simulink model "BD_PAR_AUTO_base_model"  (Simulink 10.3)
settings: Solver=ode1  StartTime=0.0  StopTime=max(cyc_mph(:,1))  FixedStep=1  MaxStep=1  RelTol=1e-3  AbsTol=1e-3
undefined symbols (not defined in the file): acc_dcdc_eff, acc_elec_eff, acc_elec_pwr, acc_mech_eff, acc_mech_pwr, acc_mech_trq, air_cp, amb_tmp, cs_charge_deplete_bool, cs_charge_trq, cs_electric_decel_spd, cs_electric_launch_spd_hi, cs_electric_launch_spd_lo, cs_hi_soc, cs_lo_soc, cs_min_trq_frac, cs_off_trq_frac, cyc_avg_time, cyc_cargo_mass, cyc_elevation_init, cyc_filter_bool, cyc_grade, cyc_mph, enable_sim_stop_distance, enable_sim_stop_max_spd, enable_sim_stop_speed, enable_sim_stop_time, enable_stop, enable_stop_fc, ess_cap_scale, ess_coulombic_eff, ess_init_soc, ess_max_ah_cap, ess_max_volts, ess_min_volts, ess_mod_airflow, ess_mod_cp, ess_mod_init_tmp, ess_module_mass, ess_module_num, ess_on, ess_r_chg, ess_r_dis, ess_res_scale_coef, ess_res_scale_fun, ess_set_tmp, ess_soc, ess_th_calc, ess_th_res_off, ess_th_res_on, ess_tmp, ess_voc, ex_calc, ex_cat_co_frac, ex_cat_ext_cp, ex_cat_ext_emisv, ex_cat_ext_init_tmp, ex_cat_ext_mass, ex_cat_ext_sarea, ex_cat_hc_frac ... (+168)
(part 12 of 15)

== system BD_PAR_AUTO_base_model/mechanical accessory loads <acc>/Mechanical Accessory Loads v2 <acc>/backward model/mechanical accessories (Nm)/Mechanical Accessories: Const Mech Var Elect/Elec Aux Loads 14V Pwr/FrontHVAC/Subsystem/Subsystem ==
  Constant1 : Constant  Value=0
  DurationOn1 : Subsystem  mask{ModelName=ModelName}
      mask prompts: ModelName "Auxiliary Load Model"
      mask init: same as BD_PAR_AUTO_base_model/electric acc loads <acc>/Electrical Accessory Loads v2 <acc>/backward model/electrical accessories (W)/Electrical Accessories: Time Variable/Elec Aux Loads 14V Pwr/ExternalLights/Subsystem/Subsystem/DurationOn1
  Hit  Crossing3 : HitCross  HitCrossingDirection=rising
  Hold Load On : RelationalOperator  Operator=<  RndMeth=Nearest  InputSameDT=on
  Hold Load On1 : RelationalOperator  RndMeth=Nearest  InputSameDT=on
  Load On : Logic  Operator=OR
  Memory5 : Memory  InitialCondition=eval('evalin(''base'',[''vinf.AuxLoads.'',ModelName,''.OnOffInfo.StartTime''])','0')
  Period1 : Subsystem  mask{ModelName=ModelName}
      mask prompts: ModelName "Auxiliary Load Model"
      mask init: same as BD_PAR_AUTO_base_model/electric acc loads <acc>/Electrical Accessory Loads v2 <acc>/backward model/electrical accessories (W)/Electrical Accessories: Time Variable/Elec Aux Loads 14V Pwr/ExternalLights/Subsystem/Subsystem/Period1
  Relational Operator1 : RelationalOperator  Operator=<=  RndMeth=Nearest  InputSameDT=on
  Relational Operator3 : RelationalOperator  Operator=>  RndMeth=Nearest  InputSameDT=on
  StartTime1 : Subsystem  mask{ModelName=ModelName}
      mask prompts: ModelName "Auxiliary Load Model"
      mask init: same as BD_PAR_AUTO_base_model/electric acc loads <acc>/Electrical Accessory Loads v2 <acc>/backward model/electrical accessories (W)/Electrical Accessories: Time Variable/Elec Aux Loads 14V Pwr/ExternalLights/Subsystem/Subsystem/StartTime1
  StartTime3 : Subsystem  mask{ModelName=ModelName}
      mask prompts: ModelName "Auxiliary Load Model"
      mask init: same as BD_PAR_AUTO_base_model/electric acc loads <acc>/Electrical Accessory Loads v2 <acc>/backward model/electrical accessories (W)/Electrical Accessories: Time Variable/Elec Aux Loads 14V Pwr/ExternalLights/Subsystem/Subsystem/StartTime1
  Sum1 : Sum  SaturateOnIntegerOverflow=on
  Sum3 : Sum  SaturateOnIntegerOverflow=on
  Switch1 : Switch  Threshold=.5
  Triggered Subsystem2 : Subsystem  TreatAsAtomicUnit=on  mask{ModelName=ModelName}
      mask prompts: ModelName "Load Name"
      mask init:
      | if (evalin('base',['isfield(vinf.AuxLoads.',ModelName,'.OnOffInfo,''StartTime'')'])); StartTime=evalin('base',['vinf.AuxLoads.',ModelName,'.OnOffInfo.StartTime']); else; StartTime=0;end
  Turn Load On : Logic  Operator=OR
  Reg Cycle On/Off : Outport
  wires:
  Memory5/1 -> Sum1/2, Sum3/2
  Sum3/1 -> Hold Load On1/2
  [time] -> Hold Load On1/1
  Turn Load On/1 -> Load On/1
  Hit  Crossing3/1 -> Turn Load On/1
  Hold Load On/1 -> Load On/2
  Hold Load On1/1 -> Turn Load On/2
  Load On/1 -> Switch1/3
  Sum1/1 -> Hold Load On/2
  [time] -> Hold Load On/1
  Relational Operator3/1 -> Hit  Crossing3/1
  [time] -> Relational Operator3/1
  StartTime1/1(Out1) -> Relational Operator3/2
  Triggered Subsystem2/1(last trig on time) -> Memory5/1
  [time] -> Triggered Subsystem2/1(time)
  Constant1/1 -> Switch1/1
  Relational Operator1/1 -> Switch1/2
  [time] -> Relational Operator1/1
  StartTime3/1(Out1) -> Relational Operator1/2
  Switch1/1 -> Reg Cycle On/Off/1, Triggered Subsystem2/Trigger
  Period1/1(Out1) -> Sum3/1
  DurationOn1/1(Out1) -> Sum1/1

== system BD_PAR_AUTO_base_model/mechanical accessory loads <acc>/Mechanical Accessory Loads v2 <acc>/backward model/mechanical accessories (Nm)/Mechanical Accessories: Const Mech Var Elect/Elec Aux Loads 14V Pwr/FrontHVAC/Subsystem/Subsystem1 ==
  Memory1 : Memory
  Memory3 : Memory
  Relational Operator1 : RelationalOperator  Operator=>  RndMeth=Nearest  InputSameDT=on
  Relational Operator2 : RelationalOperator  Operator=~=  RndMeth=Nearest  InputSameDT=on
  Sum : Sum  Inputs=+  SaturateOnIntegerOverflow=on
  ToggleTimes : Subsystem  mask{ModelName=ModelName}
      mask prompts: ModelName "Auxiliary Load Model"
      mask init: same as BD_PAR_AUTO_base_model/electric acc loads <acc>/Electrical Accessory Loads v2 <acc>/backward model/electrical accessories (W)/Electrical Accessories: Time Variable/Elec Aux Loads 14V Pwr/ExternalLights/Subsystem/Subsystem1/ToggleTimes
  Triggered Subsystem1 : Subsystem  TreatAsAtomicUnit=on  mask{ModelName=ModelName}
      mask prompts: ModelName "Load Name"
      mask init:
      | if (evalin('base',['isfield(vinf.AuxLoads.',ModelName,'.OnOffInfo,''InitialOn'')'])); InitialOn=evalin('base',['vinf.AuxLoads.',ModelName,'.OnOffInfo.InitialOn']);else;InitialOn=0;end
  Toggle On/Off : Outport
  wires:
  [time] -> Relational Operator1/1
  ToggleTimes/1(Out1) -> Relational Operator1/2
  Relational Operator1/1 -> Sum/1
  Sum/1 -> Memory1/1, Relational Operator2/1
  Relational Operator2/1 -> Triggered Subsystem1/Enable
  Triggered Subsystem1/1(Out1) -> Memory3/1, Toggle On/Off/1
  Memory3/1 -> Triggered Subsystem1/1(In1)
  Memory1/1 -> Relational Operator2/2

== system BD_PAR_AUTO_base_model/mechanical accessory loads <acc>/Mechanical Accessory Loads v2 <acc>/backward model/mechanical accessories (Nm)/Mechanical Accessories: Const Mech Var Elect/Elec Aux Loads 14V Pwr/FrontWipers/Subsystem/Subsystem ==
  Constant1 : Constant  Value=0
  DurationOn1 : Subsystem  mask{ModelName=ModelName}
      mask prompts: ModelName "Auxiliary Load Model"
      mask init: same as BD_PAR_AUTO_base_model/electric acc loads <acc>/Electrical Accessory Loads v2 <acc>/backward model/electrical accessories (W)/Electrical Accessories: Time Variable/Elec Aux Loads 14V Pwr/ExternalLights/Subsystem/Subsystem/DurationOn1
  Hit  Crossing3 : HitCross  HitCrossingDirection=rising
  Hold Load On : RelationalOperator  Operator=<  RndMeth=Nearest  InputSameDT=on
  Hold Load On1 : RelationalOperator  RndMeth=Nearest  InputSameDT=on
  Load On : Logic  Operator=OR
  Memory5 : Memory  InitialCondition=eval('evalin(''base'',[''vinf.AuxLoads.'',ModelName,''.OnOffInfo.StartTime''])','0')
  Period1 : Subsystem  mask{ModelName=ModelName}
      mask prompts: ModelName "Auxiliary Load Model"
      mask init: same as BD_PAR_AUTO_base_model/electric acc loads <acc>/Electrical Accessory Loads v2 <acc>/backward model/electrical accessories (W)/Electrical Accessories: Time Variable/Elec Aux Loads 14V Pwr/ExternalLights/Subsystem/Subsystem/Period1
  Relational Operator1 : RelationalOperator  Operator=<=  RndMeth=Nearest  InputSameDT=on
  Relational Operator3 : RelationalOperator  Operator=>  RndMeth=Nearest  InputSameDT=on
  StartTime1 : Subsystem  mask{ModelName=ModelName}
      mask prompts: ModelName "Auxiliary Load Model"
      mask init: same as BD_PAR_AUTO_base_model/electric acc loads <acc>/Electrical Accessory Loads v2 <acc>/backward model/electrical accessories (W)/Electrical Accessories: Time Variable/Elec Aux Loads 14V Pwr/ExternalLights/Subsystem/Subsystem/StartTime1
  StartTime3 : Subsystem  mask{ModelName=ModelName}
      mask prompts: ModelName "Auxiliary Load Model"
      mask init: same as BD_PAR_AUTO_base_model/electric acc loads <acc>/Electrical Accessory Loads v2 <acc>/backward model/electrical accessories (W)/Electrical Accessories: Time Variable/Elec Aux Loads 14V Pwr/ExternalLights/Subsystem/Subsystem/StartTime1
  Sum1 : Sum  SaturateOnIntegerOverflow=on
  Sum3 : Sum  SaturateOnIntegerOverflow=on
  Switch1 : Switch  Threshold=.5
  Triggered Subsystem2 : Subsystem  TreatAsAtomicUnit=on  mask{ModelName=ModelName}
      mask prompts: ModelName "Load Name"
      mask init:
      | if (evalin('base',['isfield(vinf.AuxLoads.',ModelName,'.OnOffInfo,''StartTime'')'])); StartTime=evalin('base',['vinf.AuxLoads.',ModelName,'.OnOffInfo.StartTime']); else; StartTime=0;end
  Turn Load On : Logic  Operator=OR
  Reg Cycle On/Off : Outport
  wires:
  Memory5/1 -> Sum1/2, Sum3/2
  Sum3/1 -> Hold Load On1/2
  [time] -> Hold Load On1/1
  Turn Load On/1 -> Load On/1
  Hit  Crossing3/1 -> Turn Load On/1
  Hold Load On/1 -> Load On/2
  Hold Load On1/1 -> Turn Load On/2
  Load On/1 -> Switch1/3
  Sum1/1 -> Hold Load On/2
  [time] -> Hold Load On/1
  Relational Operator3/1 -> Hit  Crossing3/1
  [time] -> Relational Operator3/1
  StartTime1/1(Out1) -> Relational Operator3/2
  Triggered Subsystem2/1(last trig on time) -> Memory5/1
  [time] -> Triggered Subsystem2/1(time)
  Constant1/1 -> Switch1/1
  Relational Operator1/1 -> Switch1/2
  [time] -> Relational Operator1/1
  StartTime3/1(Out1) -> Relational Operator1/2
  Switch1/1 -> Reg Cycle On/Off/1, Triggered Subsystem2/Trigger
  Period1/1(Out1) -> Sum3/1
  DurationOn1/1(Out1) -> Sum1/1

== system BD_PAR_AUTO_base_model/mechanical accessory loads <acc>/Mechanical Accessory Loads v2 <acc>/backward model/mechanical accessories (Nm)/Mechanical Accessories: Const Mech Var Elect/Elec Aux Loads 14V Pwr/FrontWipers/Subsystem/Subsystem1 ==
  Memory1 : Memory
  Memory3 : Memory
  Relational Operator1 : RelationalOperator  Operator=>  RndMeth=Nearest  InputSameDT=on
  Relational Operator2 : RelationalOperator  Operator=~=  RndMeth=Nearest  InputSameDT=on
  Sum : Sum  Inputs=+  SaturateOnIntegerOverflow=on
  ToggleTimes : Subsystem  mask{ModelName=ModelName}
      mask prompts: ModelName "Auxiliary Load Model"
      mask init: same as BD_PAR_AUTO_base_model/electric acc loads <acc>/Electrical Accessory Loads v2 <acc>/backward model/electrical accessories (W)/Electrical Accessories: Time Variable/Elec Aux Loads 14V Pwr/ExternalLights/Subsystem/Subsystem1/ToggleTimes
  Triggered Subsystem1 : Subsystem  TreatAsAtomicUnit=on  mask{ModelName=ModelName}
      mask prompts: ModelName "Load Name"
      mask init:
      | if (evalin('base',['isfield(vinf.AuxLoads.',ModelName,'.OnOffInfo,''InitialOn'')'])); InitialOn=evalin('base',['vinf.AuxLoads.',ModelName,'.OnOffInfo.InitialOn']);else;InitialOn=0;end
  Toggle On/Off : Outport
  wires:
  [time] -> Relational Operator1/1
  ToggleTimes/1(Out1) -> Relational Operator1/2
  Relational Operator1/1 -> Sum/1
  Sum/1 -> Memory1/1, Relational Operator2/1
  Relational Operator2/1 -> Triggered Subsystem1/Enable
  Triggered Subsystem1/1(Out1) -> Memory3/1, Toggle On/Off/1
  Memory3/1 -> Triggered Subsystem1/1(In1)
  Memory1/1 -> Relational Operator2/2

== system BD_PAR_AUTO_base_model/mechanical accessory loads <acc>/Mechanical Accessory Loads v2 <acc>/backward model/mechanical accessories (Nm)/Mechanical Accessories: Const Mech Var Elect/Elec Aux Loads 14V Pwr/HeatedSeats/Subsystem/Subsystem ==
  Constant1 : Constant  Value=0
  DurationOn1 : Subsystem  mask{ModelName=ModelName}
      mask prompts: ModelName "Auxiliary Load Model"
      mask init: same as BD_PAR_AUTO_base_model/electric acc loads <acc>/Electrical Accessory Loads v2 <acc>/backward model/electrical accessories (W)/Electrical Accessories: Time Variable/Elec Aux Loads 14V Pwr/ExternalLights/Subsystem/Subsystem/DurationOn1
  Hit  Crossing3 : HitCross  HitCrossingDirection=rising
  Hold Load On : RelationalOperator  Operator=<  RndMeth=Nearest  InputSameDT=on
  Hold Load On1 : RelationalOperator  RndMeth=Nearest  InputSameDT=on
  Load On : Logic  Operator=OR
  Memory5 : Memory  InitialCondition=eval('evalin(''base'',[''vinf.AuxLoads.'',ModelName,''.OnOffInfo.StartTime''])','0')
  Period1 : Subsystem  mask{ModelName=ModelName}
      mask prompts: ModelName "Auxiliary Load Model"
      mask init: same as BD_PAR_AUTO_base_model/electric acc loads <acc>/Electrical Accessory Loads v2 <acc>/backward model/electrical accessories (W)/Electrical Accessories: Time Variable/Elec Aux Loads 14V Pwr/ExternalLights/Subsystem/Subsystem/Period1
  Relational Operator1 : RelationalOperator  Operator=<=  RndMeth=Nearest  InputSameDT=on
  Relational Operator3 : RelationalOperator  Operator=>  RndMeth=Nearest  InputSameDT=on
  StartTime1 : Subsystem  mask{ModelName=ModelName}
      mask prompts: ModelName "Auxiliary Load Model"
      mask init: same as BD_PAR_AUTO_base_model/electric acc loads <acc>/Electrical Accessory Loads v2 <acc>/backward model/electrical accessories (W)/Electrical Accessories: Time Variable/Elec Aux Loads 14V Pwr/ExternalLights/Subsystem/Subsystem/StartTime1
  StartTime3 : Subsystem  mask{ModelName=ModelName}
      mask prompts: ModelName "Auxiliary Load Model"
      mask init: same as BD_PAR_AUTO_base_model/electric acc loads <acc>/Electrical Accessory Loads v2 <acc>/backward model/electrical accessories (W)/Electrical Accessories: Time Variable/Elec Aux Loads 14V Pwr/ExternalLights/Subsystem/Subsystem/StartTime1
  Sum1 : Sum  SaturateOnIntegerOverflow=on
  Sum3 : Sum  SaturateOnIntegerOverflow=on
  Switch1 : Switch  Threshold=.5
  Triggered Subsystem2 : Subsystem  TreatAsAtomicUnit=on  mask{ModelName=ModelName}
      mask prompts: ModelName "Load Name"
      mask init:
      | if (evalin('base',['isfield(vinf.AuxLoads.',ModelName,'.OnOffInfo,''StartTime'')'])); StartTime=evalin('base',['vinf.AuxLoads.',ModelName,'.OnOffInfo.StartTime']); else; StartTime=0;end
  Turn Load On : Logic  Operator=OR
  Reg Cycle On/Off : Outport
  wires:
  Memory5/1 -> Sum1/2, Sum3/2
  Sum3/1 -> Hold Load On1/2
  [time] -> Hold Load On1/1
  Turn Load On/1 -> Load On/1
  Hit  Crossing3/1 -> Turn Load On/1
  Hold Load On/1 -> Load On/2
  Hold Load On1/1 -> Turn Load On/2
  Load On/1 -> Switch1/3
  Sum1/1 -> Hold Load On/2
  [time] -> Hold Load On/1
  Relational Operator3/1 -> Hit  Crossing3/1
  [time] -> Relational Operator3/1
  StartTime1/1(Out1) -> Relational Operator3/2
  Triggered Subsystem2/1(last trig on time) -> Memory5/1
  [time] -> Triggered Subsystem2/1(time)
  Constant1/1 -> Switch1/1
  Relational Operator1/1 -> Switch1/2
  [time] -> Relational Operator1/1
  StartTime3/1(Out1) -> Relational Operator1/2
  Switch1/1 -> Reg Cycle On/Off/1, Triggered Subsystem2/Trigger
  Period1/1(Out1) -> Sum3/1
  DurationOn1/1(Out1) -> Sum1/1

== system BD_PAR_AUTO_base_model/mechanical accessory loads <acc>/Mechanical Accessory Loads v2 <acc>/backward model/mechanical accessories (Nm)/Mechanical Accessories: Const Mech Var Elect/Elec Aux Loads 14V Pwr/HeatedSeats/Subsystem/Subsystem1 ==
  Memory1 : Memory
  Memory3 : Memory
  Relational Operator1 : RelationalOperator  Operator=>  RndMeth=Nearest  InputSameDT=on
  Relational Operator2 : RelationalOperator  Operator=~=  RndMeth=Nearest  InputSameDT=on
  Sum : Sum  Inputs=+  SaturateOnIntegerOverflow=on
  ToggleTimes : Subsystem  mask{ModelName=ModelName}
      mask prompts: ModelName "Auxiliary Load Model"
      mask init: same as BD_PAR_AUTO_base_model/electric acc loads <acc>/Electrical Accessory Loads v2 <acc>/backward model/electrical accessories (W)/Electrical Accessories: Time Variable/Elec Aux Loads 14V Pwr/ExternalLights/Subsystem/Subsystem1/ToggleTimes
  Triggered Subsystem1 : Subsystem  TreatAsAtomicUnit=on  mask{ModelName=ModelName}
      mask prompts: ModelName "Load Name"
      mask init:
      | if (evalin('base',['isfield(vinf.AuxLoads.',ModelName,'.OnOffInfo,''InitialOn'')'])); InitialOn=evalin('base',['vinf.AuxLoads.',ModelName,'.OnOffInfo.InitialOn']);else;InitialOn=0;end
  Toggle On/Off : Outport
  wires:
  [time] -> Relational Operator1/1
  ToggleTimes/1(Out1) -> Relational Operator1/2
  Relational Operator1/1 -> Sum/1
  Sum/1 -> Memory1/1, Relational Operator2/1
  Relational Operator2/1 -> Triggered Subsystem1/Enable
  Triggered Subsystem1/1(Out1) -> Memory3/1, Toggle On/Off/1
  Memory3/1 -> Triggered Subsystem1/1(In1)
  Memory1/1 -> Relational Operator2/2

== system BD_PAR_AUTO_base_model/mechanical accessory loads <acc>/Mechanical Accessory Loads v2 <acc>/backward model/mechanical accessories (Nm)/Mechanical Accessories: Const Mech Var Elect/Elec Aux Loads 14V Pwr/RadiatorCoolingFan/Subsystem/Subsystem ==
  Constant1 : Constant  Value=0
  DurationOn1 : Subsystem  mask{ModelName=ModelName}
      mask prompts: ModelName "Auxiliary Load Model"
      mask init: same as BD_PAR_AUTO_base_model/electric acc loads <acc>/Electrical Accessory Loads v2 <acc>/backward model/electrical accessories (W)/Electrical Accessories: Time Variable/Elec Aux Loads 14V Pwr/ExternalLights/Subsystem/Subsystem/DurationOn1
  Hit  Crossing3 : HitCross  HitCrossingDirection=rising
  Hold Load On : RelationalOperator  Operator=<  RndMeth=Nearest  InputSameDT=on
  Hold Load On1 : RelationalOperator  RndMeth=Nearest  InputSameDT=on
  Load On : Logic  Operator=OR
  Memory5 : Memory  InitialCondition=eval('evalin(''base'',[''vinf.AuxLoads.'',ModelName,''.OnOffInfo.StartTime''])','0')
  Period1 : Subsystem  mask{ModelName=ModelName}
      mask prompts: ModelName "Auxiliary Load Model"
      mask init: same as BD_PAR_AUTO_base_model/electric acc loads <acc>/Electrical Accessory Loads v2 <acc>/backward model/electrical accessories (W)/Electrical Accessories: Time Variable/Elec Aux Loads 14V Pwr/ExternalLights/Subsystem/Subsystem/Period1
  Relational Operator1 : RelationalOperator  Operator=<=  RndMeth=Nearest  InputSameDT=on
  Relational Operator3 : RelationalOperator  Operator=>  RndMeth=Nearest  InputSameDT=on
  StartTime1 : Subsystem  mask{ModelName=ModelName}
      mask prompts: ModelName "Auxiliary Load Model"
      mask init: same as BD_PAR_AUTO_base_model/electric acc loads <acc>/Electrical Accessory Loads v2 <acc>/backward model/electrical accessories (W)/Electrical Accessories: Time Variable/Elec Aux Loads 14V Pwr/ExternalLights/Subsystem/Subsystem/StartTime1
  StartTime3 : Subsystem  mask{ModelName=ModelName}
      mask prompts: ModelName "Auxiliary Load Model"
      mask init: same as BD_PAR_AUTO_base_model/electric acc loads <acc>/Electrical Accessory Loads v2 <acc>/backward model/electrical accessories (W)/Electrical Accessories: Time Variable/Elec Aux Loads 14V Pwr/ExternalLights/Subsystem/Subsystem/StartTime1
  Sum1 : Sum  SaturateOnIntegerOverflow=on
  Sum3 : Sum  SaturateOnIntegerOverflow=on
  Switch1 : Switch  Threshold=.5
  Triggered Subsystem2 : Subsystem  TreatAsAtomicUnit=on  mask{ModelName=ModelName}
      mask prompts: ModelName "Load Name"
      mask init:
      | if (evalin('base',['isfield(vinf.AuxLoads.',ModelName,'.OnOffInfo,''StartTime'')'])); StartTime=evalin('base',['vinf.AuxLoads.',ModelName,'.OnOffInfo.StartTime']); else; StartTime=0;end
  Turn Load On : Logic  Operator=OR
  Reg Cycle On/Off : Outport
  wires:
  Memory5/1 -> Sum1/2, Sum3/2
  Sum3/1 -> Hold Load On1/2
  [time] -> Hold Load On1/1
  Turn Load On/1 -> Load On/1
  Hit  Crossing3/1 -> Turn Load On/1
  Hold Load On/1 -> Load On/2
  Hold Load On1/1 -> Turn Load On/2
  Load On/1 -> Switch1/3
  Sum1/1 -> Hold Load On/2
  [time] -> Hold Load On/1
  Relational Operator3/1 -> Hit  Crossing3/1
  [time] -> Relational Operator3/1
  StartTime1/1(Out1) -> Relational Operator3/2
  Triggered Subsystem2/1(last trig on time) -> Memory5/1
  [time] -> Triggered Subsystem2/1(time)
  Constant1/1 -> Switch1/1
  Relational Operator1/1 -> Switch1/2
  [time] -> Relational Operator1/1
  StartTime3/1(Out1) -> Relational Operator1/2
  Switch1/1 -> Reg Cycle On/Off/1, Triggered Subsystem2/Trigger
  Period1/1(Out1) -> Sum3/1
  DurationOn1/1(Out1) -> Sum1/1

== system BD_PAR_AUTO_base_model/mechanical accessory loads <acc>/Mechanical Accessory Loads v2 <acc>/backward model/mechanical accessories (Nm)/Mechanical Accessories: Const Mech Var Elect/Elec Aux Loads 14V Pwr/RadiatorCoolingFan/Subsystem/Subsystem1 ==
  Memory1 : Memory
  Memory3 : Memory
  Relational Operator1 : RelationalOperator  Operator=>  RndMeth=Nearest  InputSameDT=on
  Relational Operator2 : RelationalOperator  Operator=~=  RndMeth=Nearest  InputSameDT=on
  Sum : Sum  Inputs=+  SaturateOnIntegerOverflow=on
  ToggleTimes : Subsystem  mask{ModelName=ModelName}
      mask prompts: ModelName "Auxiliary Load Model"
      mask init: same as BD_PAR_AUTO_base_model/electric acc loads <acc>/Electrical Accessory Loads v2 <acc>/backward model/electrical accessories (W)/Electrical Accessories: Time Variable/Elec Aux Loads 14V Pwr/ExternalLights/Subsystem/Subsystem1/ToggleTimes
  Triggered Subsystem1 : Subsystem  TreatAsAtomicUnit=on  mask{ModelName=ModelName}
      mask prompts: ModelName "Load Name"
      mask init:
      | if (evalin('base',['isfield(vinf.AuxLoads.',ModelName,'.OnOffInfo,''InitialOn'')'])); InitialOn=evalin('base',['vinf.AuxLoads.',ModelName,'.OnOffInfo.InitialOn']);else;InitialOn=0;end
  Toggle On/Off : Outport
  wires:
  [time] -> Relational Operator1/1
  ToggleTimes/1(Out1) -> Relational Operator1/2
  Relational Operator1/1 -> Sum/1
  Sum/1 -> Memory1/1, Relational Operator2/1
  Relational Operator2/1 -> Triggered Subsystem1/Enable
  Triggered Subsystem1/1(Out1) -> Memory3/1, Toggle On/Off/1
  Memory3/1 -> Triggered Subsystem1/1(In1)
  Memory1/1 -> Relational Operator2/2

== system BD_PAR_AUTO_base_model/mechanical accessory loads <acc>/Mechanical Accessory Loads v2 <acc>/backward model/mechanical accessories (Nm)/Mechanical Accessories: Const Mech Var Elect/Elec Aux Loads 14V Pwr/Radio/Subsystem/Subsystem ==
  Constant1 : Constant  Value=0
  DurationOn1 : Subsystem  mask{ModelName=ModelName}
      mask prompts: ModelName "Auxiliary Load Model"
      mask init: same as BD_PAR_AUTO_base_model/electric acc loads <acc>/Electrical Accessory Loads v2 <acc>/backward model/electrical accessories (W)/Electrical Accessories: Time Variable/Elec Aux Loads 14V Pwr/ExternalLights/Subsystem/Subsystem/DurationOn1
  Hit  Crossing3 : HitCross  HitCrossingDirection=rising
  Hold Load On : RelationalOperator  Operator=<  RndMeth=Nearest  InputSameDT=on
  Hold Load On1 : RelationalOperator  RndMeth=Nearest  InputSameDT=on
  Load On : Logic  Operator=OR
  Memory5 : Memory  InitialCondition=eval('evalin(''base'',[''vinf.AuxLoads.'',ModelName,''.OnOffInfo.StartTime''])','0')
  Period1 : Subsystem  mask{ModelName=ModelName}
      mask prompts: ModelName "Auxiliary Load Model"
      mask init: same as BD_PAR_AUTO_base_model/electric acc loads <acc>/Electrical Accessory Loads v2 <acc>/backward model/electrical accessories (W)/Electrical Accessories: Time Variable/Elec Aux Loads 14V Pwr/ExternalLights/Subsystem/Subsystem/Period1
  Relational Operator1 : RelationalOperator  Operator=<=  RndMeth=Nearest  InputSameDT=on
  Relational Operator3 : RelationalOperator  Operator=>  RndMeth=Nearest  InputSameDT=on
  StartTime1 : Subsystem  mask{ModelName=ModelName}
      mask prompts: ModelName "Auxiliary Load Model"
      mask init: same as BD_PAR_AUTO_base_model/electric acc loads <acc>/Electrical Accessory Loads v2 <acc>/backward model/electrical accessories (W)/Electrical Accessories: Time Variable/Elec Aux Loads 14V Pwr/ExternalLights/Subsystem/Subsystem/StartTime1
  StartTime3 : Subsystem  mask{ModelName=ModelName}
      mask prompts: ModelName "Auxiliary Load Model"
      mask init: same as BD_PAR_AUTO_base_model/electric acc loads <acc>/Electrical Accessory Loads v2 <acc>/backward model/electrical accessories (W)/Electrical Accessories: Time Variable/Elec Aux Loads 14V Pwr/ExternalLights/Subsystem/Subsystem/StartTime1
  Sum1 : Sum  SaturateOnIntegerOverflow=on
  Sum3 : Sum  SaturateOnIntegerOverflow=on
  Switch1 : Switch  Threshold=.5
  Triggered Subsystem2 : Subsystem  TreatAsAtomicUnit=on  mask{ModelName=ModelName}
      mask prompts: ModelName "Load Name"
      mask init:
      | if (evalin('base',['isfield(vinf.AuxLoads.',ModelName,'.OnOffInfo,''StartTime'')'])); StartTime=evalin('base',['vinf.AuxLoads.',ModelName,'.OnOffInfo.StartTime']); else; StartTime=0;end
  Turn Load On : Logic  Operator=OR
  Reg Cycle On/Off : Outport
  wires:
  Memory5/1 -> Sum1/2, Sum3/2
  Sum3/1 -> Hold Load On1/2
  [time] -> Hold Load On1/1
  Turn Load On/1 -> Load On/1
  Hit  Crossing3/1 -> Turn Load On/1
  Hold Load On/1 -> Load On/2
  Hold Load On1/1 -> Turn Load On/2
  Load On/1 -> Switch1/3
  Sum1/1 -> Hold Load On/2
  [time] -> Hold Load On/1
  Relational Operator3/1 -> Hit  Crossing3/1
  [time] -> Relational Operator3/1
  StartTime1/1(Out1) -> Relational Operator3/2
  Triggered Subsystem2/1(last trig on time) -> Memory5/1
  [time] -> Triggered Subsystem2/1(time)
  Constant1/1 -> Switch1/1
  Relational Operator1/1 -> Switch1/2
  [time] -> Relational Operator1/1
  StartTime3/1(Out1) -> Relational Operator1/2
  Switch1/1 -> Reg Cycle On/Off/1, Triggered Subsystem2/Trigger
  Period1/1(Out1) -> Sum3/1
  DurationOn1/1(Out1) -> Sum1/1

== system BD_PAR_AUTO_base_model/mechanical accessory loads <acc>/Mechanical Accessory Loads v2 <acc>/backward model/mechanical accessories (Nm)/Mechanical Accessories: Const Mech Var Elect/Elec Aux Loads 14V Pwr/Radio/Subsystem/Subsystem1 ==
  Memory1 : Memory
  Memory3 : Memory
  Relational Operator1 : RelationalOperator  Operator=>  RndMeth=Nearest  InputSameDT=on
  Relational Operator2 : RelationalOperator  Operator=~=  RndMeth=Nearest  InputSameDT=on
  Sum : Sum  Inputs=+  SaturateOnIntegerOverflow=on
  ToggleTimes : Subsystem  mask{ModelName=ModelName}
      mask prompts: ModelName "Auxiliary Load Model"
      mask init: same as BD_PAR_AUTO_base_model/electric acc loads <acc>/Electrical Accessory Loads v2 <acc>/backward model/electrical accessories (W)/Electrical Accessories: Time Variable/Elec Aux Loads 14V Pwr/ExternalLights/Subsystem/Subsystem1/ToggleTimes
  Triggered Subsystem1 : Subsystem  TreatAsAtomicUnit=on  mask{ModelName=ModelName}
      mask prompts: ModelName "Load Name"
      mask init:
      | if (evalin('base',['isfield(vinf.AuxLoads.',ModelName,'.OnOffInfo,''InitialOn'')'])); InitialOn=evalin('base',['vinf.AuxLoads.',ModelName,'.OnOffInfo.InitialOn']);else;InitialOn=0;end
  Toggle On/Off : Outport
  wires:
  [time] -> Relational Operator1/1
  ToggleTimes/1(Out1) -> Relational Operator1/2
  Relational Operator1/1 -> Sum/1
  Sum/1 -> Memory1/1, Relational Operator2/1
  Relational Operator2/1 -> Triggered Subsystem1/Enable
  Triggered Subsystem1/1(Out1) -> Memory3/1, Toggle On/Off/1
  Memory3/1 -> Triggered Subsystem1/1(In1)
  Memory1/1 -> Relational Operator2/2

== system BD_PAR_AUTO_base_model/mechanical accessory loads <acc>/Mechanical Accessory Loads v2 <acc>/backward model/mechanical accessories (Nm)/Mechanical Accessories: Const Mech Var Elect/Elec Aux Loads 14V Pwr/RearDefrost/Subsystem/Subsystem ==
  Constant1 : Constant  Value=0
  DurationOn1 : Subsystem  mask{ModelName=ModelName}
      mask prompts: ModelName "Auxiliary Load Model"
      mask init: same as BD_PAR_AUTO_base_model/electric acc loads <acc>/Electrical Accessory Loads v2 <acc>/backward model/electrical accessories (W)/Electrical Accessories: Time Variable/Elec Aux Loads 14V Pwr/ExternalLights/Subsystem/Subsystem/DurationOn1
  Hit  Crossing3 : HitCross  HitCrossingDirection=rising
  Hold Load On : RelationalOperator  Operator=<  RndMeth=Nearest  InputSameDT=on
  Hold Load On1 : RelationalOperator  RndMeth=Nearest  InputSameDT=on
  Load On : Logic  Operator=OR
  Memory5 : Memory  InitialCondition=eval('evalin(''base'',[''vinf.AuxLoads.'',ModelName,''.OnOffInfo.StartTime''])','0')
  Period1 : Subsystem  mask{ModelName=ModelName}
      mask prompts: ModelName "Auxiliary Load Model"
      mask init: same as BD_PAR_AUTO_base_model/electric acc loads <acc>/Electrical Accessory Loads v2 <acc>/backward model/electrical accessories (W)/Electrical Accessories: Time Variable/Elec Aux Loads 14V Pwr/ExternalLights/Subsystem/Subsystem/Period1
  Relational Operator1 : RelationalOperator  Operator=<=  RndMeth=Nearest  InputSameDT=on
  Relational Operator3 : RelationalOperator  Operator=>  RndMeth=Nearest  InputSameDT=on
  StartTime1 : Subsystem  mask{ModelName=ModelName}
      mask prompts: ModelName "Auxiliary Load Model"
      mask init: same as BD_PAR_AUTO_base_model/electric acc loads <acc>/Electrical Accessory Loads v2 <acc>/backward model/electrical accessories (W)/Electrical Accessories: Time Variable/Elec Aux Loads 14V Pwr/ExternalLights/Subsystem/Subsystem/StartTime1
  StartTime3 : Subsystem  mask{ModelName=ModelName}
      mask prompts: ModelName "Auxiliary Load Model"
      mask init: same as BD_PAR_AUTO_base_model/electric acc loads <acc>/Electrical Accessory Loads v2 <acc>/backward model/electrical accessories (W)/Electrical Accessories: Time Variable/Elec Aux Loads 14V Pwr/ExternalLights/Subsystem/Subsystem/StartTime1
  Sum1 : Sum  SaturateOnIntegerOverflow=on
  Sum3 : Sum  SaturateOnIntegerOverflow=on
  Switch1 : Switch  Threshold=.5
  Triggered Subsystem2 : Subsystem  TreatAsAtomicUnit=on  mask{ModelName=ModelName}
      mask prompts: ModelName "Load Name"
      mask init:
      | if (evalin('base',['isfield(vinf.AuxLoads.',ModelName,'.OnOffInfo,''StartTime'')'])); StartTime=evalin('base',['vinf.AuxLoads.',ModelName,'.OnOffInfo.StartTime']); else; StartTime=0;end
  Turn Load On : Logic  Operator=OR
  Reg Cycle On/Off : Outport
  wires:
  Memory5/1 -> Sum1/2, Sum3/2
  Sum3/1 -> Hold Load On1/2
  [time] -> Hold Load On1/1
  Turn Load On/1 -> Load On/1
  Hit  Crossing3/1 -> Turn Load On/1
  Hold Load On/1 -> Load On/2
  Hold Load On1/1 -> Turn Load On/2
  Load On/1 -> Switch1/3
  Sum1/1 -> Hold Load On/2
  [time] -> Hold Load On/1
  Relational Operator3/1 -> Hit  Crossing3/1
  [time] -> Relational Operator3/1
  StartTime1/1(Out1) -> Relational Operator3/2
  Triggered Subsystem2/1(last trig on time) -> Memory5/1
  [time] -> Triggered Subsystem2/1(time)
  Constant1/1 -> Switch1/1
  Relational Operator1/1 -> Switch1/2
  [time] -> Relational Operator1/1
  StartTime3/1(Out1) -> Relational Operator1/2
  Switch1/1 -> Reg Cycle On/Off/1, Triggered Subsystem2/Trigger
  Period1/1(Out1) -> Sum3/1
  DurationOn1/1(Out1) -> Sum1/1

== system BD_PAR_AUTO_base_model/mechanical accessory loads <acc>/Mechanical Accessory Loads v2 <acc>/backward model/mechanical accessories (Nm)/Mechanical Accessories: Const Mech Var Elect/Elec Aux Loads 14V Pwr/RearDefrost/Subsystem/Subsystem1 ==
  Memory1 : Memory
  Memory3 : Memory
  Relational Operator1 : RelationalOperator  Operator=>  RndMeth=Nearest  InputSameDT=on
  Relational Operator2 : RelationalOperator  Operator=~=  RndMeth=Nearest  InputSameDT=on
  Sum : Sum  Inputs=+  SaturateOnIntegerOverflow=on
  ToggleTimes : Subsystem  mask{ModelName=ModelName}
      mask prompts: ModelName "Auxiliary Load Model"
      mask init: same as BD_PAR_AUTO_base_model/electric acc loads <acc>/Electrical Accessory Loads v2 <acc>/backward model/electrical accessories (W)/Electrical Accessories: Time Variable/Elec Aux Loads 14V Pwr/ExternalLights/Subsystem/Subsystem1/ToggleTimes
  Triggered Subsystem1 : Subsystem  TreatAsAtomicUnit=on  mask{ModelName=ModelName}
      mask prompts: ModelName "Load Name"
      mask init:
      | if (evalin('base',['isfield(vinf.AuxLoads.',ModelName,'.OnOffInfo,''InitialOn'')'])); InitialOn=evalin('base',['vinf.AuxLoads.',ModelName,'.OnOffInfo.InitialOn']);else;InitialOn=0;end
  Toggle On/Off : Outport
  wires:
  [time] -> Relational Operator1/1
  ToggleTimes/1(Out1) -> Relational Operator1/2
  Relational Operator1/1 -> Sum/1
  Sum/1 -> Memory1/1, Relational Operator2/1
  Relational Operator2/1 -> Triggered Subsystem1/Enable
  Triggered Subsystem1/1(Out1) -> Memory3/1, Toggle On/Off/1
  Memory3/1 -> Triggered Subsystem1/1(In1)
  Memory1/1 -> Relational Operator2/2

== system BD_PAR_AUTO_base_model/mechanical accessory loads <acc>/Mechanical Accessory Loads v2 <acc>/backward model/mechanical accessories (Nm)/Mechanical Accessories: Const Mech Var Elect/Elec Aux Loads 14V Pwr/RearHVAC/Subsystem/Subsystem ==
  Constant1 : Constant  Value=0
  DurationOn1 : Subsystem  mask{ModelName=ModelName}
      mask prompts: ModelName "Auxiliary Load Model"
      mask init: same as BD_PAR_AUTO_base_model/electric acc loads <acc>/Electrical Accessory Loads v2 <acc>/backward model/electrical accessories (W)/Electrical Accessories: Time Variable/Elec Aux Loads 14V Pwr/ExternalLights/Subsystem/Subsystem/DurationOn1
  Hit  Crossing3 : HitCross  HitCrossingDirection=rising
  Hold Load On : RelationalOperator  Operator=<  RndMeth=Nearest  InputSameDT=on
  Hold Load On1 : RelationalOperator  RndMeth=Nearest  InputSameDT=on
  Load On : Logic  Operator=OR
  Memory5 : Memory  InitialCondition=eval('evalin(''base'',[''vinf.AuxLoads.'',ModelName,''.OnOffInfo.StartTime''])','0')
  Period1 : Subsystem  mask{ModelName=ModelName}
      mask prompts: ModelName "Auxiliary Load Model"
      mask init: same as BD_PAR_AUTO_base_model/electric acc loads <acc>/Electrical Accessory Loads v2 <acc>/backward model/electrical accessories (W)/Electrical Accessories: Time Variable/Elec Aux Loads 14V Pwr/ExternalLights/Subsystem/Subsystem/Period1
  Relational Operator1 : RelationalOperator  Operator=<=  RndMeth=Nearest  InputSameDT=on
  Relational Operator3 : RelationalOperator  Operator=>  RndMeth=Nearest  InputSameDT=on
  StartTime1 : Subsystem  mask{ModelName=ModelName}
      mask prompts: ModelName "Auxiliary Load Model"
      mask init: same as BD_PAR_AUTO_base_model/electric acc loads <acc>/Electrical Accessory Loads v2 <acc>/backward model/electrical accessories (W)/Electrical Accessories: Time Variable/Elec Aux Loads 14V Pwr/ExternalLights/Subsystem/Subsystem/StartTime1
  StartTime3 : Subsystem  mask{ModelName=ModelName}
      mask prompts: ModelName "Auxiliary Load Model"
      mask init: same as BD_PAR_AUTO_base_model/electric acc loads <acc>/Electrical Accessory Loads v2 <acc>/backward model/electrical accessories (W)/Electrical Accessories: Time Variable/Elec Aux Loads 14V Pwr/ExternalLights/Subsystem/Subsystem/StartTime1
  Sum1 : Sum  SaturateOnIntegerOverflow=on
  Sum3 : Sum  SaturateOnIntegerOverflow=on
  Switch1 : Switch  Threshold=.5
  Triggered Subsystem2 : Subsystem  TreatAsAtomicUnit=on  mask{ModelName=ModelName}
      mask prompts: ModelName "Load Name"
      mask init:
      | if (evalin('base',['isfield(vinf.AuxLoads.',ModelName,'.OnOffInfo,''StartTime'')'])); StartTime=evalin('base',['vinf.AuxLoads.',ModelName,'.OnOffInfo.StartTime']); else; StartTime=0;end
  Turn Load On : Logic  Operator=OR
  Reg Cycle On/Off : Outport
  wires:
  Memory5/1 -> Sum1/2, Sum3/2
  Sum3/1 -> Hold Load On1/2
  [time] -> Hold Load On1/1
  Turn Load On/1 -> Load On/1
  Hit  Crossing3/1 -> Turn Load On/1
  Hold Load On/1 -> Load On/2
  Hold Load On1/1 -> Turn Load On/2
  Load On/1 -> Switch1/3
  Sum1/1 -> Hold Load On/2
  [time] -> Hold Load On/1
  Relational Operator3/1 -> Hit  Crossing3/1
  [time] -> Relational Operator3/1
  StartTime1/1(Out1) -> Relational Operator3/2
  Triggered Subsystem2/1(last trig on time) -> Memory5/1
  [time] -> Triggered Subsystem2/1(time)
  Constant1/1 -> Switch1/1
  Relational Operator1/1 -> Switch1/2
  [time] -> Relational Operator1/1
  StartTime3/1(Out1) -> Relational Operator1/2
  Switch1/1 -> Reg Cycle On/Off/1, Triggered Subsystem2/Trigger
  Period1/1(Out1) -> Sum3/1
  DurationOn1/1(Out1) -> Sum1/1

== system BD_PAR_AUTO_base_model/mechanical accessory loads <acc>/Mechanical Accessory Loads v2 <acc>/backward model/mechanical accessories (Nm)/Mechanical Accessories: Const Mech Var Elect/Elec Aux Loads 14V Pwr/RearHVAC/Subsystem/Subsystem1 ==
  Memory1 : Memory
  Memory3 : Memory
  Relational Operator1 : RelationalOperator  Operator=>  RndMeth=Nearest  InputSameDT=on
  Relational Operator2 : RelationalOperator  Operator=~=  RndMeth=Nearest  InputSameDT=on
  Sum : Sum  Inputs=+  SaturateOnIntegerOverflow=on
  ToggleTimes : Subsystem  mask{ModelName=ModelName}
      mask prompts: ModelName "Auxiliary Load Model"
      mask init: same as BD_PAR_AUTO_base_model/electric acc loads <acc>/Electrical Accessory Loads v2 <acc>/backward model/electrical accessories (W)/Electrical Accessories: Time Variable/Elec Aux Loads 14V Pwr/ExternalLights/Subsystem/Subsystem1/ToggleTimes
  Triggered Subsystem1 : Subsystem  TreatAsAtomicUnit=on  mask{ModelName=ModelName}
      mask prompts: ModelName "Load Name"
      mask init:
      | if (evalin('base',['isfield(vinf.AuxLoads.',ModelName,'.OnOffInfo,''InitialOn'')'])); InitialOn=evalin('base',['vinf.AuxLoads.',ModelName,'.OnOffInfo.InitialOn']);else;InitialOn=0;end
  Toggle On/Off : Outport
  wires:
  [time] -> Relational Operator1/1
  ToggleTimes/1(Out1) -> Relational Operator1/2
  Relational Operator1/1 -> Sum/1
  Sum/1 -> Memory1/1, Relational Operator2/1
  Relational Operator2/1 -> Triggered Subsystem1/Enable
  Triggered Subsystem1/1(Out1) -> Memory3/1, Toggle On/Off/1
  Memory3/1 -> Triggered Subsystem1/1(In1)
  Memory1/1 -> Relational Operator2/2

== system BD_PAR_AUTO_base_model/mechanical accessory loads <acc>/Mechanical Accessory Loads v2 <acc>/backward model/mechanical accessories (Nm)/Mechanical Accessories: Const Mech Var Elect/Elec Aux Loads 14V Pwr/RearWipers/Subsystem/Subsystem ==
  Constant1 : Constant  Value=0
  DurationOn1 : Subsystem  mask{ModelName=ModelName}
      mask prompts: ModelName "Auxiliary Load Model"
      mask init: same as BD_PAR_AUTO_base_model/electric acc loads <acc>/Electrical Accessory Loads v2 <acc>/backward model/electrical accessories (W)/Electrical Accessories: Time Variable/Elec Aux Loads 14V Pwr/ExternalLights/Subsystem/Subsystem/DurationOn1
  Hit  Crossing3 : HitCross  HitCrossingDirection=rising
  Hold Load On : RelationalOperator  Operator=<  RndMeth=Nearest  InputSameDT=on
  Hold Load On1 : RelationalOperator  RndMeth=Nearest  InputSameDT=on
  Load On : Logic  Operator=OR
  Memory5 : Memory  InitialCondition=eval('evalin(''base'',[''vinf.AuxLoads.'',ModelName,''.OnOffInfo.StartTime''])','0')
  Period1 : Subsystem  mask{ModelName=ModelName}
      mask prompts: ModelName "Auxiliary Load Model"
      mask init: same as BD_PAR_AUTO_base_model/electric acc loads <acc>/Electrical Accessory Loads v2 <acc>/backward model/electrical accessories (W)/Electrical Accessories: Time Variable/Elec Aux Loads 14V Pwr/ExternalLights/Subsystem/Subsystem/Period1
  Relational Operator1 : RelationalOperator  Operator=<=  RndMeth=Nearest  InputSameDT=on
  Relational Operator3 : RelationalOperator  Operator=>  RndMeth=Nearest  InputSameDT=on
  StartTime1 : Subsystem  mask{ModelName=ModelName}
      mask prompts: ModelName "Auxiliary Load Model"
      mask init: same as BD_PAR_AUTO_base_model/electric acc loads <acc>/Electrical Accessory Loads v2 <acc>/backward model/electrical accessories (W)/Electrical Accessories: Time Variable/Elec Aux Loads 14V Pwr/ExternalLights/Subsystem/Subsystem/StartTime1
  StartTime3 : Subsystem  mask{ModelName=ModelName}
      mask prompts: ModelName "Auxiliary Load Model"
      mask init: same as BD_PAR_AUTO_base_model/electric acc loads <acc>/Electrical Accessory Loads v2 <acc>/backward model/electrical accessories (W)/Electrical Accessories: Time Variable/Elec Aux Loads 14V Pwr/ExternalLights/Subsystem/Subsystem/StartTime1
  Sum1 : Sum  SaturateOnIntegerOverflow=on
  Sum3 : Sum  SaturateOnIntegerOverflow=on
  Switch1 : Switch  Threshold=.5
  Triggered Subsystem2 : Subsystem  TreatAsAtomicUnit=on  mask{ModelName=ModelName}
      mask prompts: ModelName "Load Name"
      mask init:
      | if (evalin('base',['isfield(vinf.AuxLoads.',ModelName,'.OnOffInfo,''StartTime'')'])); StartTime=evalin('base',['vinf.AuxLoads.',ModelName,'.OnOffInfo.StartTime']); else; StartTime=0;end
  Turn Load On : Logic  Operator=OR
  Reg Cycle On/Off : Outport
  wires:
  Memory5/1 -> Sum1/2, Sum3/2
  Sum3/1 -> Hold Load On1/2
  [time] -> Hold Load On1/1
  Turn Load On/1 -> Load On/1
  Hit  Crossing3/1 -> Turn Load On/1
  Hold Load On/1 -> Load On/2
  Hold Load On1/1 -> Turn Load On/2
  Load On/1 -> Switch1/3
  Sum1/1 -> Hold Load On/2
  [time] -> Hold Load On/1
  Relational Operator3/1 -> Hit  Crossing3/1
  [time] -> Relational Operator3/1
  StartTime1/1(Out1) -> Relational Operator3/2
  Triggered Subsystem2/1(last trig on time) -> Memory5/1
  [time] -> Triggered Subsystem2/1(time)
  Constant1/1 -> Switch1/1
  Relational Operator1/1 -> Switch1/2
  [time] -> Relational Operator1/1
  StartTime3/1(Out1) -> Relational Operator1/2
  Switch1/1 -> Reg Cycle On/Off/1, Triggered Subsystem2/Trigger
  Period1/1(Out1) -> Sum3/1
  DurationOn1/1(Out1) -> Sum1/1

== system BD_PAR_AUTO_base_model/mechanical accessory loads <acc>/Mechanical Accessory Loads v2 <acc>/backward model/mechanical accessories (Nm)/Mechanical Accessories: Const Mech Var Elect/Elec Aux Loads 14V Pwr/RearWipers/Subsystem/Subsystem1 ==
  Memory1 : Memory
  Memory3 : Memory
  Relational Operator1 : RelationalOperator  Operator=>  RndMeth=Nearest  InputSameDT=on
  Relational Operator2 : RelationalOperator  Operator=~=  RndMeth=Nearest  InputSameDT=on
  Sum : Sum  Inputs=+  SaturateOnIntegerOverflow=on
  ToggleTimes : Subsystem  mask{ModelName=ModelName}
      mask prompts: ModelName "Auxiliary Load Model"
      mask init: same as BD_PAR_AUTO_base_model/electric acc loads <acc>/Electrical Accessory Loads v2 <acc>/backward model/electrical accessories (W)/Electrical Accessories: Time Variable/Elec Aux Loads 14V Pwr/ExternalLights/Subsystem/Subsystem1/ToggleTimes
  Triggered Subsystem1 : Subsystem  TreatAsAtomicUnit=on  mask{ModelName=ModelName}
      mask prompts: ModelName "Load Name"
      mask init:
      | if (evalin('base',['isfield(vinf.AuxLoads.',ModelName,'.OnOffInfo,''InitialOn'')'])); InitialOn=evalin('base',['vinf.AuxLoads.',ModelName,'.OnOffInfo.InitialOn']);else;InitialOn=0;end
  Toggle On/Off : Outport
  wires:
  [time] -> Relational Operator1/1
  ToggleTimes/1(Out1) -> Relational Operator1/2
  Relational Operator1/1 -> Sum/1
  Sum/1 -> Memory1/1, Relational Operator2/1
  Relational Operator2/1 -> Triggered Subsystem1/Enable
  Triggered Subsystem1/1(Out1) -> Memory3/1, Toggle On/Off/1
  Memory3/1 -> Triggered Subsystem1/1(In1)
  Memory1/1 -> Relational Operator2/2

== system BD_PAR_AUTO_base_model/mechanical accessory loads <acc>/Mechanical Accessory Loads v2 <acc>/backward model/mechanical accessories (Nm)/Mechanical Accessories: Const Mech Var Elect/Elec Aux Loads 14V Pwr/Starter/Starter/Subsystem ==
  In1 : Inport
  In2 : Inport  Port=2
  Constant : Constant  Value=vinf.AuxLoads.Starter.DurationOn
  Constant1 : Constant  Value=0
  Constant2 : Constant
  Last Engine On Time : Subsystem  TreatAsAtomicUnit=on
  Relational Operator : RelationalOperator  Operator=>  RndMeth=Nearest  InputSameDT=on
  Sum : Sum  Inputs=-+  SaturateOnIntegerOverflow=on
  Switch : Switch  Threshold=.5
  Out1 : Outport
  wires:
  Constant/1 -> Relational Operator/1
  Sum/1 -> Relational Operator/2
  In2/1 -> Sum/2, Last Engine On Time/1(In1)  "Current TIme"
  Last Engine On Time/1(Out1) -> Sum/1
  Relational Operator/1 -> Switch/2
  Constant1/1 -> Switch/3
  In1/1 -> Last Engine On Time/Trigger
  Constant2/1 -> Switch/1
  Switch/1 -> Out1/1

== system BD_PAR_AUTO_base_model/mechanical accessory loads <acc>/Mechanical Accessory Loads v2 <acc>/backward model/mechanical accessories (Nm)/Mechanical Accessories: Const Mech Var Elect/Elec Aux Loads 14V Pwr/TurnSignals/Subsystem/Subsystem ==
  Constant1 : Constant  Value=0
  DurationOn1 : Subsystem  mask{ModelName=ModelName}
      mask prompts: ModelName "Auxiliary Load Model"
      mask init: same as BD_PAR_AUTO_base_model/electric acc loads <acc>/Electrical Accessory Loads v2 <acc>/backward model/electrical accessories (W)/Electrical Accessories: Time Variable/Elec Aux Loads 14V Pwr/ExternalLights/Subsystem/Subsystem/DurationOn1
  Hit  Crossing3 : HitCross  HitCrossingDirection=rising
  Hold Load On : RelationalOperator  Operator=<  RndMeth=Nearest  InputSameDT=on
  Hold Load On1 : RelationalOperator  RndMeth=Nearest  InputSameDT=on
  Load On : Logic  Operator=OR
  Memory5 : Memory  InitialCondition=eval('evalin(''base'',[''vinf.AuxLoads.'',ModelName,''.OnOffInfo.StartTime''])','0')
  Period1 : Subsystem  mask{ModelName=ModelName}
      mask prompts: ModelName "Auxiliary Load Model"
      mask init: same as BD_PAR_AUTO_base_model/electric acc loads <acc>/Electrical Accessory Loads v2 <acc>/backward model/electrical accessories (W)/Electrical Accessories: Time Variable/Elec Aux Loads 14V Pwr/ExternalLights/Subsystem/Subsystem/Period1
  Relational Operator1 : RelationalOperator  Operator=<=  RndMeth=Nearest  InputSameDT=on
  Relational Operator3 : RelationalOperator  Operator=>  RndMeth=Nearest  InputSameDT=on
  StartTime1 : Subsystem  mask{ModelName=ModelName}
      mask prompts: ModelName "Auxiliary Load Model"
      mask init: same as BD_PAR_AUTO_base_model/electric acc loads <acc>/Electrical Accessory Loads v2 <acc>/backward model/electrical accessories (W)/Electrical Accessories: Time Variable/Elec Aux Loads 14V Pwr/ExternalLights/Subsystem/Subsystem/StartTime1
  StartTime3 : Subsystem  mask{ModelName=ModelName}
      mask prompts: ModelName "Auxiliary Load Model"
      mask init: same as BD_PAR_AUTO_base_model/electric acc loads <acc>/Electrical Accessory Loads v2 <acc>/backward model/electrical accessories (W)/Electrical Accessories: Time Variable/Elec Aux Loads 14V Pwr/ExternalLights/Subsystem/Subsystem/StartTime1
  Sum1 : Sum  SaturateOnIntegerOverflow=on
  Sum3 : Sum  SaturateOnIntegerOverflow=on
  Switch1 : Switch  Threshold=.5
  Triggered Subsystem2 : Subsystem  TreatAsAtomicUnit=on  mask{ModelName=ModelName}
      mask prompts: ModelName "Load Name"
      mask init:
      | if (evalin('base',['isfield(vinf.AuxLoads.',ModelName,'.OnOffInfo,''StartTime'')'])); StartTime=evalin('base',['vinf.AuxLoads.',ModelName,'.OnOffInfo.StartTime']); else; StartTime=0;end
  Turn Load On : Logic  Operator=OR
  Reg Cycle On/Off : Outport
  wires:
  Memory5/1 -> Sum1/2, Sum3/2
  Sum3/1 -> Hold Load On1/2
  [time] -> Hold Load On1/1
  Turn Load On/1 -> Load On/1
  Hit  Crossing3/1 -> Turn Load On/1
  Hold Load On/1 -> Load On/2
  Hold Load On1/1 -> Turn Load On/2
  Load On/1 -> Switch1/3
  Sum1/1 -> Hold Load On/2
  [time] -> Hold Load On/1
  Relational Operator3/1 -> Hit  Crossing3/1
  [time] -> Relational Operator3/1
  StartTime1/1(Out1) -> Relational Operator3/2
  Triggered Subsystem2/1(last trig on time) -> Memory5/1
  [time] -> Triggered Subsystem2/1(time)
  Constant1/1 -> Switch1/1
  Relational Operator1/1 -> Switch1/2
  [time] -> Relational Operator1/1
  StartTime3/1(Out1) -> Relational Operator1/2
  Switch1/1 -> Reg Cycle On/Off/1, Triggered Subsystem2/Trigger
  Period1/1(Out1) -> Sum3/1
  DurationOn1/1(Out1) -> Sum1/1

== system BD_PAR_AUTO_base_model/mechanical accessory loads <acc>/Mechanical Accessory Loads v2 <acc>/backward model/mechanical accessories (Nm)/Mechanical Accessories: Const Mech Var Elect/Elec Aux Loads 14V Pwr/TurnSignals/Subsystem/Subsystem1 ==
  Memory1 : Memory
  Memory3 : Memory
  Relational Operator1 : RelationalOperator  Operator=>  RndMeth=Nearest  InputSameDT=on
  Relational Operator2 : RelationalOperator  Operator=~=  RndMeth=Nearest  InputSameDT=on
  Sum : Sum  Inputs=+  SaturateOnIntegerOverflow=on
  ToggleTimes : Subsystem  mask{ModelName=ModelName}
      mask prompts: ModelName "Auxiliary Load Model"
      mask init: same as BD_PAR_AUTO_base_model/electric acc loads <acc>/Electrical Accessory Loads v2 <acc>/backward model/electrical accessories (W)/Electrical Accessories: Time Variable/Elec Aux Loads 14V Pwr/ExternalLights/Subsystem/Subsystem1/ToggleTimes
  Triggered Subsystem1 : Subsystem  TreatAsAtomicUnit=on  mask{ModelName=ModelName}
      mask prompts: ModelName "Load Name"
      mask init:
      | if (evalin('base',['isfield(vinf.AuxLoads.',ModelName,'.OnOffInfo,''InitialOn'')'])); InitialOn=evalin('base',['vinf.AuxLoads.',ModelName,'.OnOffInfo.InitialOn']);else;InitialOn=0;end
  Toggle On/Off : Outport
  wires:
  [time] -> Relational Operator1/1
  ToggleTimes/1(Out1) -> Relational Operator1/2
  Relational Operator1/1 -> Sum/1
  Sum/1 -> Memory1/1, Relational Operator2/1
  Relational Operator2/1 -> Triggered Subsystem1/Enable
  Triggered Subsystem1/1(Out1) -> Memory3/1, Toggle On/Off/1
  Memory3/1 -> Triggered Subsystem1/1(In1)
  Memory1/1 -> Relational Operator2/2
